simulink model "OutputToContinuousStimAndVisualization"  (R2016b)
settings: Solver=FixedStepDiscrete  StartTime=0.0  StopTime=inf  FixedStep=sCoreParams.core.stepPeriod  RelTol=1e-3  EnableMultiTasking=on
undefined symbols (not defined in the file or in its folder): sCoreParams
libraries: dspswit3 x4
settings Model: DataTypeOverride=Double  MinMaxOverflowLogging=ForceOff  Creator=rzelmann  LastModifiedBy=rzelmann
settings SolverCC: EnableConcurrentExecution=on  ConcurrentTasks=on  AutoInsertRateTranBlk=on
settings DataIOCC: SaveFormat=StructureWithTime  SaveOutput=off  SignalLogging=off  DSMLogging=off  SaveTime=off
settings OptimizationCC: BlockReduction=off  DefaultParameterBehavior=Inlined  LifeSpan=inf
settings DebuggingCC: AllowSymbolicDim=off  SFUnexpectedBacktrackingDiag=warning  SFNoUnconditionalDefaultTransitionDiag=warning  SFExecutionAtInitializationDiag=none
settings HardwareCC: ProdBitPerPointer=32  ProdBitPerSizeT=32  ProdBitPerPtrDiffT=32  ProdLargestAtomicFloat=None  ProdWordSize=32  ProdLongLongMode=on  ProdHWDeviceType=Generic->32-bit x86 compatible
settings ModelReferenceCC: UpdateModelReferenceTargets=Force  ParallelModelReferenceMATLABWorkerInit=Load Top Model  ModelReferenceNumInstancesAllowed=Single  ModelReferencePassRootInputsByReference=off
settings RTWCC: SystemTargetFile=slrt.tlc  TemplateMakefile=slrt_default_tmf  Description=Simulink Real-Time  RTWCompilerOptimization=on
settings CodeAppCC: MaxIdLength=63
settings TargetCC: CodeReplacementLibrary=XPC_BLAS  ParMdlRefBuildCompliant=on  ConcurrentExecutionCompliant=on  GeneratePreprocessorConditionals=Use local settings  MatFileLogging=on  MATLABClassNameForMDSCustomization=xpcAperiodicCustomization
settings ConfigComp: CovMetricSettings=dw  CovHtmlReporting=on  CovSaveCumulativeToWorkspaceVar=on  CovSaveSingleToWorkspaceVar=on  CovExternalEMLEnable=off

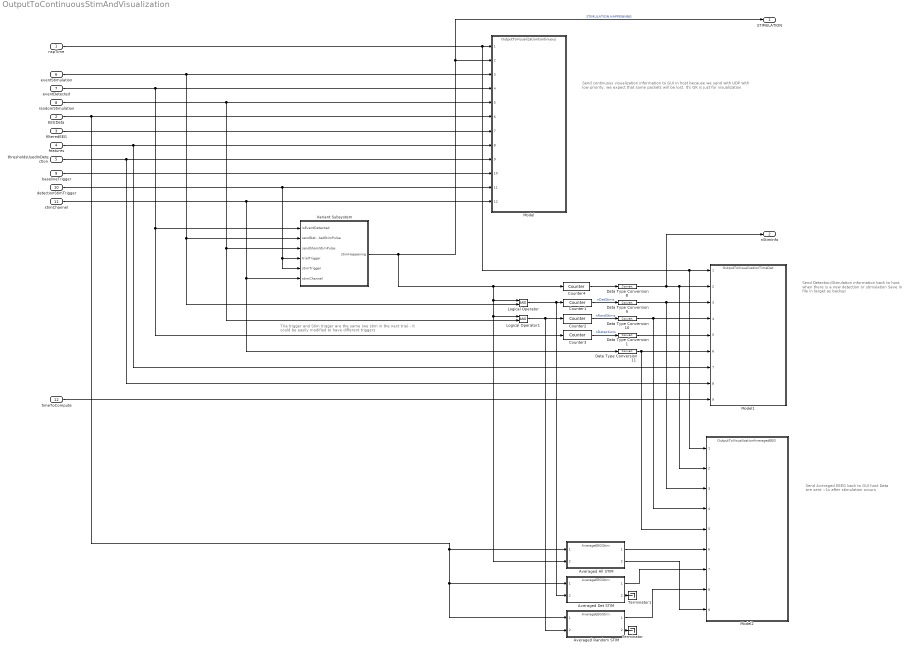
== system OutputToContinuousStimAndVisualization ==
  note: Send Averaged EEEG back to GUI host
      | Data are sent ~1s after stimulation occurs
  note: Send Detection/Stmulation information back to host
      |  when there is a new detection or stimulation
      | Save in file in target as backup
  note: Send continuous visualization information to GUI in host
      | because we send with UDP with low priority, we expect that some packets will be lost.
      | It's OK is just for visualization
  note: Tria trigger and Stim trigger are the same (we stim in the next tria)
      | - it could be easily modified to have different triggers
  nspTime : Inport  SampleTime=sCoreParams.core.stepPeriod
  EEGData : Inport  Port=2  SampleTime=sCoreParams.core.stepPeriod
  filteredEEG : Inport  Port=3  SampleTime=sCoreParams.core.stepPeriod
  features : Inport  Port=4  SampleTime=sCoreParams.core.stepPeriod
  thresholdsUsedInDetection : Inport  Port=5  SampleTime=sCoreParams.core.stepPeriod
  eventStimulation : Inport  Port=6  SampleTime=sCoreParams.core.stepPeriod
  eventDetected : Inport  Port=7  SampleTime=sCoreParams.core.stepPeriod
  randomStimulation : Inport  Port=8  SampleTime=sCoreParams.core.stepPeriod
  baselineTrigger : Inport  Port=9  SampleTime=sCoreParams.core.stepPeriod
  detectionStimTrigger : Inport  Port=10  SampleTime=sCoreParams.core.stepPeriod
  stimChannel : Inport  Port=11  SampleTime=sCoreParams.core.stepPeriod
  timeToCompute : Inport  Port=12  OutDataTypeStr=boolean  SampleTime=sCoreParams.core.stepPeriod
  Averaged All STIM : ModelReference  ModelNameDialog=AverageEEGStim.slx  SimulationMode=Normal  ModelReferenceVersion=1.332
  Averaged Det STIM : ModelReference  ModelNameDialog=AverageEEGStim.slx  SimulationMode=Normal  ModelReferenceVersion=1.332
  Averaged Random STIM : ModelReference  ModelNameDialog=AverageEEGStim.slx  SimulationMode=Normal  ModelReferenceVersion=1.332
  Counter{1..4} (4 alike) : dspswit3/Counter  Direction=Up  CountEvent=Rising edge  CounterSize=User defined  MaxCount=1024  InitialCount=0  Output=Count  HitValue=32  ResetInput=off  SamplesPerFrame=1  Ts=1  CntDtype=int32  HitDtype=Logical
  Data Type Conversion{1,8..11} (5 alike) : DataTypeConversion
  Logical Operator : Logic  IconShape=distinctive  AllPortsSameDT=off  OutDataTypeStr=boolean
  Logical Operator1 : Logic  IconShape=distinctive  AllPortsSameDT=off  OutDataTypeStr=boolean
  Model : ModelReference  ModelNameDialog=OutputToVisualizationContinuous.slx  SimulationMode=Normal  ModelReferenceVersion=1.308
  Model1 : ModelReference  ModelNameDialog=OutputToVisualizationTimeDet.slx  SimulationMode=Normal  ModelReferenceVersion=1.293
  Model2 : ModelReference  ModelNameDialog=OutputToVisualizationAveragedEEG.slx  SimulationMode=Normal  ModelReferenceVersion=1.308
  Terminator : Terminator
  Terminator1 : Terminator
  Variant Subsystem : Subsystem  Variant=on
  STIMULATION : Outport
  nStimInfo : Outport  Port=2
  wires:
  Counter1/1 -> Data Type Conversion9/1  "nDetStims"
  nspTime/1 -> Model2/1, Model1/1, Model/1
  Data Type Conversion11/1 -> Model2/5, Model1/6
  Variant Subsystem/1(stimHappening) -> Model/2, STIMULATION/1, Averaged All STIM/2, Logical Operator1/1, Logical Operator/1, Counter4/1  "STIMULATION HAPPENNING"
  Logical Operator1/1 -> Averaged Random STIM/2, Counter2/1
  detectionStimTrigger/1 -> Model/11, Variant Subsystem/5(stimTrigger), Variant Subsystem/4(trialTrigger)
  stimChannel/1 -> Model/12, Variant Subsystem/6(stimChannel), Data Type Conversion11/1
  Logical Operator/1 -> Averaged Det STIM/2, Counter1/1
  Counter2/1 -> Data Type Conversion10/1  "nRandStims"
  randomStimulation/1 -> Model/5, Variant Subsystem/3(sendShamStimPulse), Logical Operator1/2
  Data Type Conversion8/1 -> nStimInfo/1, Model2/2, Model1/2
  eventStimulation/1 -> Model/3, Variant Subsystem/2(sendDetectedStimPulse), Logical Operator/2
  Counter4/1 -> Data Type Conversion8/1
  EEGData/1 -> Averaged Random STIM/1, Averaged Det STIM/1, Averaged All STIM/1, Model/6
  filteredEEG/1 -> Model/7
  eventDetected/1 -> Variant Subsystem/1(isEventDetected), Counter3/1, Model/4
  baselineTrigger/1 -> Model/10
  features/1 -> Model1/7, Model/8
  thresholdsUsedInDetection/1 -> Model1/8, Model/9
  Data Type Conversion9/1 -> Model2/3, Model1/3
  Data Type Conversion10/1 -> Model2/4, Model1/4
  Counter3/1 -> Data Type Conversion1/1  "nDetections"
  Data Type Conversion1/1 -> Model1/5
  timeToCompute/1 -> Model1/9
  Averaged All STIM/1 -> Model2/6
  Averaged Det STIM/1 -> Model2/7
  Averaged Random STIM/1 -> Model2/8
  Averaged Det STIM/2 -> Terminator1/1
  Averaged Random STIM/2 -> Terminator/1
  Averaged All STIM/2 -> Model2/9

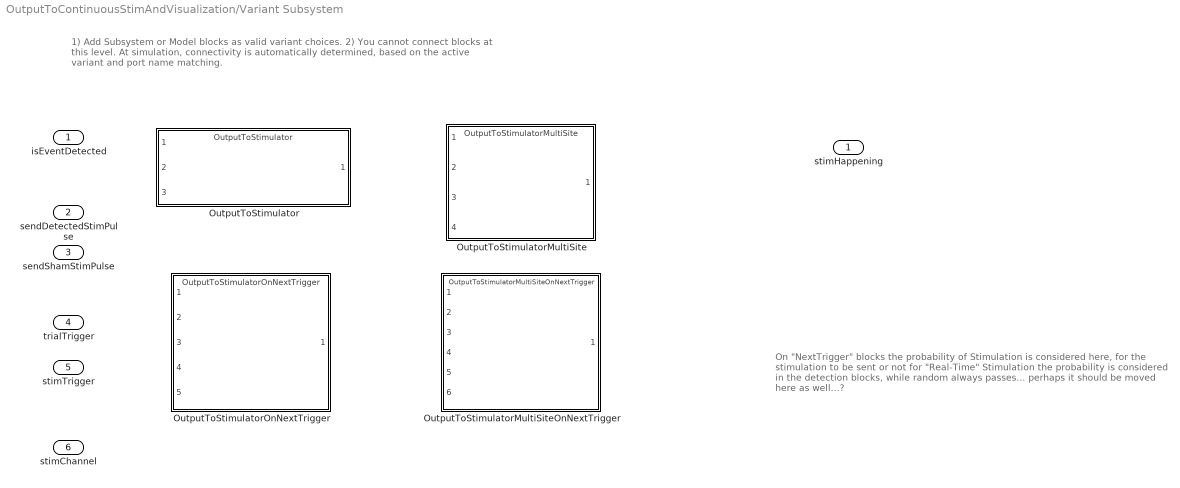
== system OutputToContinuousStimAndVisualization/Variant Subsystem ==
  note: On "NextTrigger" blocks the probability of Stimulation is considered here,
      | for the stimulation to be sent or not
      | for "Real-Time" Stimulation the probability is considered in the detection blocks,
      | while random always passes... perhaps it should be moved here as well...?
  note: 1) Add Subsystem or Model blocks as valid variant choices.
      | 2) You cannot connect blocks at this level. At simulation, connectivity is automatically
      | determined, based on the active variant and port name matching.
  isEventDetected : Inport
  sendDetectedStimPulse : Inport  Port=2
  sendShamStimPulse : Inport  Port=3
  trialTrigger : Inport  Port=4
  stimTrigger : Inport  Port=5
  stimChannel : Inport  Port=6  OutDataTypeStr=int32
  OutputToStimulator : ModelReference  ModelNameDialog=OutputToStimulator  SimulationMode=Normal  VariantControl=variantParams_STIMULATION_REALTIME  ModelReferenceVersion=1.34
  OutputToStimulatorMultiSite : ModelReference  ModelNameDialog=OutputToStimulatorMultiSite.slx  SimulationMode=Normal  VariantControl=variantParams_STIMULATION_MULTISITE_REALTIME  ModelReferenceVersion=1.46
  OutputToStimulatorMultiSiteOnNextTrigger : ModelReference  ModelNameDialog=OutputToStimulatorMultiSiteOnNextTrigger.slx  SimulationMode=Normal  VariantControl=variantParams_STIMULATION_MULTISITE_NEXTTRIGGER  ModelReferenceVersion=1.78
  OutputToStimulatorOnNextTrigger : ModelReference  ModelNameDialog=OutputToStimulatorOnNextTrigger  SimulationMode=Normal  VariantControl=variantParams_STIMULATION_ONNEXTTRIGGER  ModelReferenceVersion=1.86
  stimHappening : Outport
